simulink model "ARDroneReplay_V3"  (R2023b)
settings: Solver=ode1  StartTime=0.0  StopTime=54.2150  FixedStep=sampleTime  RelTol=1e-3
values from neighbouring files (symbols this model uses):
  meanAcce3 = [-0.0108248998661285 0.149142386085094 -9.620196316402833]    [initialize_paper.m]
  P0 = diag([0.01, 0.01, 0.01, 0.01, 0.01, 0.01])    [initialize_paper.m]
  Sigma = diag([0.05, 0.05, 0.05, 0.00001, 0.00001, 0.00001])    [initialize_paper.m]
  Theta = diag([0.05,0.05,0.05])    [initialize_paper.m]
undefined symbols (not defined in the file or in its folder): sampleTime
libraries: ARBlocks x2
settings Model: ExtModeTrigDuration=100000  Creator=Paul  LastModifiedBy=André
settings SolverCC: AlgebraicLoopSolver=TrustRegion  AutoInsertRateTranBlk=on
settings DataIOCC: LimitDataPoints=on  SaveFormat=Array  SignalLoggingSaveFormat=ModelDataLogs  ReturnWorkspaceOutputs=off  TimeSaveName=time
settings OptimizationCC: ExpressionDepthLimit=2147483647  InitFltsAndDblsToZero=on
settings DebuggingCC: UnderspecifiedInitializationDetection=Classic  MergeDetectMultiDrivingBlocksExec=none  SolverPrmCheckMsg=warning  FcnCallInpInsideContextMsg=warning  UnconnectedInputMsg=warning  UnconnectedOutputMsg=warning  UnconnectedLineMsg=warning  StateNameClashWarn=warning  SFUnexpectedBacktrackingDiag=warning  SFNoUnconditionalDefaultTransitionDiag=warning  SFExecutionAtInitializationDiag=none  ArithmeticOperatorsInVariantConditions=warning
settings HardwareCC: ProdBitPerLong=64  ProdHWDeviceType=Intel->x86-64 (Linux 64)
settings ModelReferenceCC: EnableRefExpFcnMdlSchedulingChecks=on  PropagateSignalLabelsOutOfModel=off
settings SFSimCC: SimUseLocalCustomCode=off  CustomCodeUndefinedFunction=UseInterfaceOnly
settings RTWCC: Description=Simulink Desktop Real-Time  SystemTargetFile=sldrt.tlc  TemplateMakefile=sldrt.tmf  RTWUseLocalCustomCode=off  RTWCompilerOptimization=on
settings CodeAppCC: MaxIdLength=95  StateflowObjectComments=on
settings SimulinkDesktopRealTimeCC: TargetLibSuffix=_sldrt.a  TargetPreCompLibLocation=C:\Program Files\MATLAB\R2023b\toolbox\sldrt\lib\win64  TargetLangStandard=C89/C90 (ANSI)  SupportVariableSizeSignals=off
settings ConfigComp: CovMetricSettings=dw  CovSaveCumulativeToWorkspaceVar=on  CovSaveSingleToWorkspaceVar=on  CovExternalEMLEnable=off

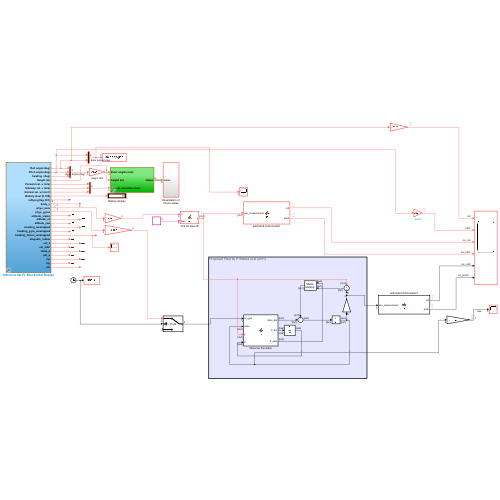
[thumbnail: Simulink's stored preview of the top-level diagram]
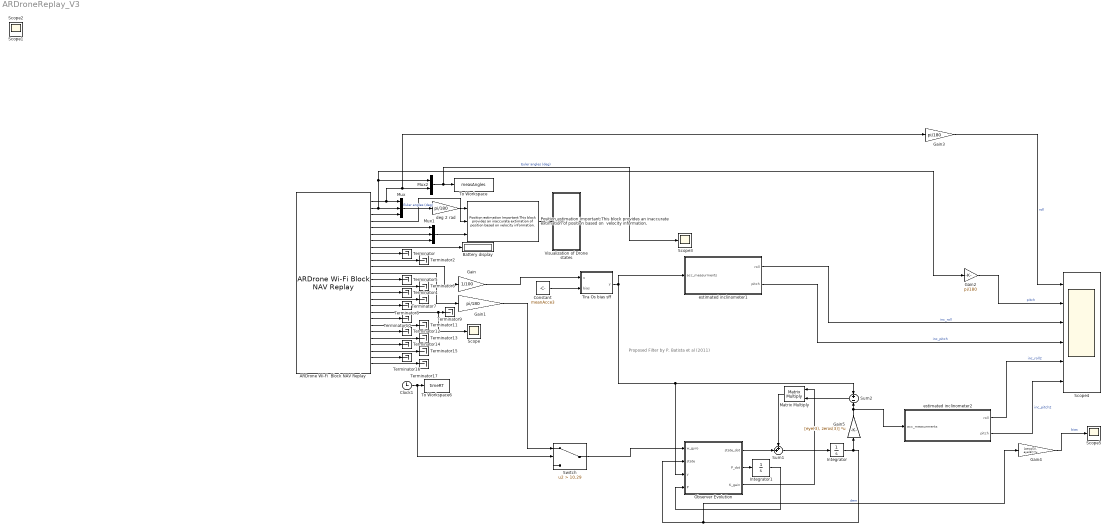
== system ARDroneReplay_V3 ==
  note: Proposed Filter by P. Batista et al (2011)
  ARDrone Wi-Fi  Block NAV Replay : ARBlocks/ARDrone Wi-Fi  Block NAV Replay  SystemSampleTime=-1  VariantActivationTime=update diagram  AllowFlexibleInterface=on  Latency=0  AutoFrameSizeCalculation=off
  Battery display : Display
  Clock1 : Clock
  Constant : Constant  Value=meanAcce3
  Gain : Gain  Gain=1/100
  Gain1 : Gain  Gain=pi/180
  Gain2 : Gain  Gain=pi/180
  Gain3 : Gain  Gain=pi/180
  Gain4 : Gain  Gain=[zeros(3), eye(3)]  Multiplication=Matrix(K*u) (u vector)
  Gain5 : Gain  Gain=[eye(3), zeros(3)]  Multiplication=Matrix(K*u) (u vector)
  Integrator : Integrator  InitialCondition=[ 0;0; -9.81 ;0.0;0.0;0.0]
  Integrator1 : Integrator  InitialCondition=P0
  Matrix Multiply : Product  Multiplication=Matrix(*)
  Mux : Mux  Inputs=3
  Mux1 : Mux  Inputs=3
  Mux2 : Mux  Inputs=2
  Observer Evolution : MATLAB Function  TreatAsAtomicUnit=on
  "Position estimation Important:This block provides an inaccurate extimation of position based on  velocity information. " : ARBlocks/Position estimation Important:This block provides an  inaccurate extimation of position  based on  velocity information.   SystemSampleTime=-1  VariantActivationTime=update diagram  AllowFlexibleInterface=on  Latency=0  AutoFrameSizeCalculation=off
  Scope{,1..3,5} (5 alike) : Scope
  Scope4 : Scope  NumInputPorts=6
  Sum1 : Sum  Inputs=++|
  Sum2 : Sum  Inputs=+|-
  Switch : Switch  Criteria=u2 > Threshold  Threshold=10.29  SaturateOnIntegerOverflow=off  InputSameDT=off
  Terminator{,2,4..17} (16 alike) : Terminator
  Tira Os bias sff : MATLAB Function  TreatAsAtomicUnit=on
  To Workspace : ToWorkspace  VariableName=measAngles  SaveFormat=Structure With Time  SampleTime=-1
  To Workspace6 : ToWorkspace  VariableName=timeRT  SampleTime=sampleTime
  Visualization of Drone states : Subsystem
  deg 2 rad : Gain  Gain=pi/180
  estimated inclinometer1 : MATLAB Function  TreatAsAtomicUnit=on
  estimated inclinometer2 : MATLAB Function  TreatAsAtomicUnit=on
  wires:
  ARDrone Wi-Fi  Block NAV Replay/1 -> Gain3/1, Mux2/2, Mux/1
  ARDrone Wi-Fi  Block NAV Replay/2 -> Mux2/1, Gain2/1, Mux/2
  ARDrone Wi-Fi  Block NAV Replay/5 -> Mux1/1
  ARDrone Wi-Fi  Block NAV Replay/6 -> Mux1/2
  ARDrone Wi-Fi  Block NAV Replay/7 -> Mux1/3
  Mux/1 -> deg 2 rad/1  "Euler angles (deg)"
  ARDrone Wi-Fi  Block NAV Replay/8 -> Battery display/1
  "Position estimation Important:This block provides an inaccurate extimation of position based on  velocity information. "/1 -> Visualization of Drone states/1(states)
  deg 2 rad/1 -> "Position estimation Important:This block provides an inaccurate extimation of position based on  velocity information. "/1
  ARDrone Wi-Fi  Block NAV Replay/4 -> "Position estimation Important:This block provides an inaccurate extimation of position based on  velocity information. "/2
  Mux1/1 -> "Position estimation Important:This block provides an inaccurate extimation of position based on  velocity information. "/3
  ARDrone Wi-Fi  Block NAV Replay/3 -> Mux/3
  ARDrone Wi-Fi  Block NAV Replay/9 -> Terminator/1
  Clock1/1 -> Switch/2, To Workspace6/1
  ARDrone Wi-Fi  Block NAV Replay/15 -> Terminator4/1
  ARDrone Wi-Fi  Block NAV Replay/10 -> Terminator2/1
  ARDrone Wi-Fi  Block NAV Replay/13 -> Terminator5/1
  ARDrone Wi-Fi  Block NAV Replay/14 -> Terminator6/1
  ARDrone Wi-Fi  Block NAV Replay/17 -> Terminator8/1
  ARDrone Wi-Fi  Block NAV Replay/16 -> Terminator7/1
  ARDrone Wi-Fi  Block NAV Replay/19 -> Terminator10/1
  ARDrone Wi-Fi  Block NAV Replay/18 -> Scope/1, Terminator9/1
  ARDrone Wi-Fi  Block NAV Replay/21 -> Terminator12/1
  ARDrone Wi-Fi  Block NAV Replay/20 -> Terminator11/1
  ARDrone Wi-Fi  Block NAV Replay/23 -> Terminator14/1
  ARDrone Wi-Fi  Block NAV Replay/22 -> Terminator13/1
  ARDrone Wi-Fi  Block NAV Replay/25 -> Terminator16/1
  ARDrone Wi-Fi  Block NAV Replay/24 -> Terminator15/1
  ARDrone Wi-Fi  Block NAV Replay/26 -> Terminator17/1
  ARDrone Wi-Fi  Block NAV Replay/11 -> Gain/1
  ARDrone Wi-Fi  Block NAV Replay/12 -> Gain1/1
  Mux2/1 -> Scope3/1, To Workspace/1  "Euler angles (deg)"
  Gain5/1 -> estimated inclinometer2/1(acc_measurments), Sum2/2
  Observer Evolution/3(K_gain) -> Matrix Multiply/1
  Sum2/1 -> Matrix Multiply/2
  Matrix Multiply/1 -> Sum1/1
  Integrator1/1 -> Observer Evolution/4(P)
  Sum1/1 -> Integrator/1
  Observer Evolution/2(P_dot) -> Integrator1/1
  Observer Evolution/1(state_dot) -> Sum1/2
  Integrator/1 -> Gain5/1, Gain4/1, Observer Evolution/2(state)  "dem"
  Gain/1 -> Tira Os bias sff/1(u)
  estimated inclinometer2/1(roll) -> Scope4/5  "inc_roll2"
  estimated inclinometer2/2(pitch) -> Scope4/6  "inc_pitch2"
  Gain2/1 -> Scope4/2  "pitch"
  Gain3/1 -> Scope4/1  "roll"
  estimated inclinometer1/1(roll) -> Scope4/3  "inc_roll"
  estimated inclinometer1/2(pitch) -> Scope4/4  "inc_pitch"
  Switch/1 -> Observer Evolution/1(w_gyro)
  Gain1/1 -> Switch/1
  Gain4/1 -> Scope5/1  "bias"
  Tira Os bias sff/1(y) -> estimated inclinometer1/1(acc_measurments), Sum2/1, Observer Evolution/3(y)
  Constant/1 -> Tira Os bias sff/2(bias)

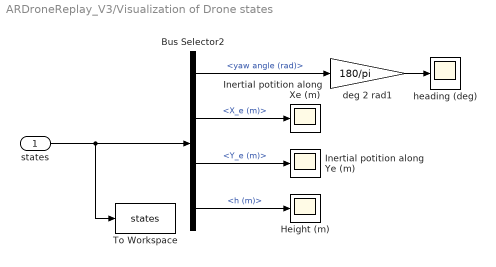
== system ARDroneReplay_V3/Visualization of Drone states ==
  states : Inport
  Bus Selector2 : BusSelector  OutputSignals=yaw angle (rad),X_e (m),Y_e (m),h (m)
  Height (m) : Scope
  Inertial potition along Xe (m) : Scope
  Inertial potition along Ye (m) : Scope
  To Workspace : ToWorkspace  VariableName=states  SaveFormat=Structure With Time  SampleTime=-1
  deg 2 rad1 : Gain  Gain=180/pi
  heading (deg) : Scope
  wires:
  states/1 -> To Workspace/1, Bus Selector2/1
  Bus Selector2/1 -> deg 2 rad1/1  "<yaw angle (rad)>"
  Bus Selector2/2 -> Inertial potition along Xe (m)/1  "<X_e (m)>"
  Bus Selector2/3 -> Inertial potition along Ye (m)/1  "<Y_e (m)>"
  Bus Selector2/4 -> Height (m)/1  "<h (m)>"
  deg 2 rad1/1 -> heading (deg)/1

== matlab function ARDroneReplay_V3/Observer Evolution ==
  data: w_gyro input; state input; y input; state_dot output; P_dot output; P input; Sigma parameter; Theta parameter; K_gain output
function [state_dot, P_dot, K_gain]= fcn(w_gyro, state,y,P, Sigma, Theta)

%y = state(1:3);
%bias = state(4:6);

C = [eye(3), zeros(3)];


skew_gyro = [0 -w_gyro(3)  w_gyro(2) ; w_gyro(3) 0 -w_gyro(1) ; -w_gyro(2) w_gyro(1) 0 ];

skew_att = [0 -y(3) y(2) ; y(3) 0 -y(1) ; -y(2) y(1) 0 ];

% build time varying matrix A
A = [-skew_gyro, -skew_att; zeros(3), zeros(3)];

state_dot = A*state;


P_dot = A*P + P*A' + Sigma - P*C'*inv(Theta)*C*P; 
K_gain = P*C'*inv(Theta); %#ok<*MINV>

== matlab function ARDroneReplay_V3/estimated inclinometer1 ==
  data: acc_measurments input; roll output; pitch output
function [roll, pitch] = fcn(acc_measurments)
ax = acc_measurments(1);
ay = acc_measurments(2);
az = acc_measurments(3);

ag = sqrt(ax*ax + ay*ay + az*az);
if ag == 0
    pitch = 0;
    roll = 0;
    return
end

roll = atan(ay/az);
pitch = asin(ax/ag);

== matlab function ARDroneReplay_V3/estimated inclinometer2 ==
  data: acc_measurments input; roll output; pitch output
function [roll, pitch] = fcn(acc_measurments)
ax = acc_measurments(1);
ay = acc_measurments(2);
az = acc_measurments(3);

ag = sqrt(ax*ax + ay*ay + az*az);
if ag == 0
    pitch = 0;
    roll = 0;
    return
end

roll = atan(ay/az);
pitch = asin(ax/ag);

== matlab function ARDroneReplay_V3/Tira Os bias sff ==
  data: u input; y output; bias input
function y = fcn(u, bias)

u(1) = u(1) - bias(1);
u(2) = u(2) - bias(2);
u(3) = u(3) - (bias(3)+9.8);

y = u;
